simulink model "kalman_trial"  (R2016b)
settings: Solver=VariableStepAuto  StartTime=0.0  StopTime=200  RelTol=1e-3
undefined symbols (not defined in the file or in its folder): F, G, H, Kf
libraries: simulink x1
settings Model: Creator=Thomas  LastModifiedBy=Thomas

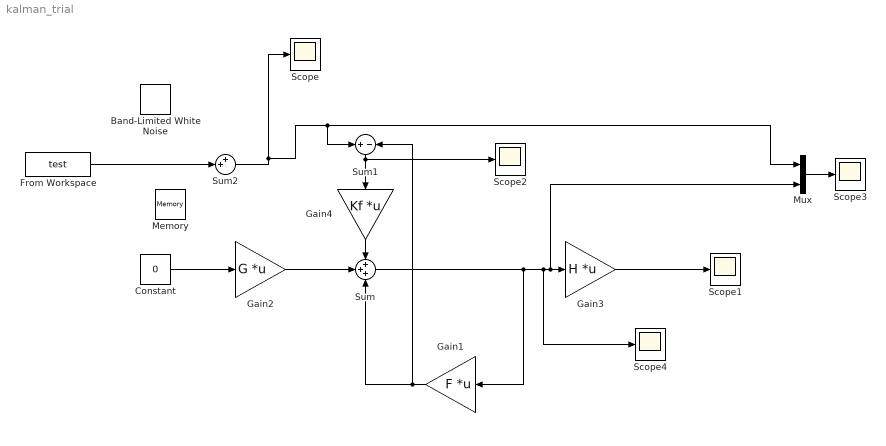
== system kalman_trial ==
  Band-Limited White Noise : simulink/Sources/Band-Limited White Noise  Cov=[0.01]  Ts=0.1  seed=[23341]
  Constant : Constant  Value=0
  From Workspace : FromWorkspace  VariableName=test  SampleTime=0
  Gain1 : Gain  Gain=F  Multiplication=Matrix(K*u)
  Gain2 : Gain  Gain=G  Multiplication=Matrix(K*u)
  Gain3 : Gain  Gain=H  Multiplication=Matrix(K*u)
  Gain4 : Gain  Gain=Kf  Multiplication=Matrix(K*u)
  Memory : Memory
  Mux : Mux  Inputs=2
  Scope{,1..4} (5 alike) : Scope
  Sum : Sum  Inputs=+++
  Sum1 : Sum  Inputs=+-
  Sum2 : Sum  Inputs=++|
  wires:
  Sum/1 -> Scope4/1, Mux/2, Gain3/1, Gain1/1
  Gain2/1 -> Sum/2
  Gain1/1 -> Sum1/2, Sum/3
  Gain4/1 -> Sum/1
  Sum1/1 -> Gain4/1, Scope2/1
  Gain3/1 -> Scope1/1
  Constant/1 -> Gain2/1
  Mux/1 -> Scope3/1
  From Workspace/1 -> Sum2/2
  Sum2/1 -> Sum1/1, Mux/1, Scope/1
